simulink model "SEIRv1"  (R2019b)
settings: Solver=VariableStepAuto  StartTime=0.0  StopTime=365  RelTol=1e-3
settings Model: Creator=Alex  LastModifiedBy=Alex

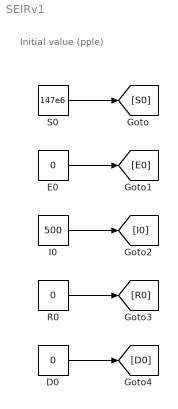
== system SEIRv1 ==
  note: Initial value (pple)
  D0 : Constant  Value=0
  E0 : Constant  Value=0
  I0 : Constant  Value=500
  R0 : Constant  Value=0
  S0 : Constant  Value=147e6
  wires:
  S0/1 -> [S0]
  E0/1 -> [E0]
  I0/1 -> [I0]
  R0/1 -> [R0]
  D0/1 -> [D0]
